simulink model "SimuOnlineComputeI1Level2C"  (R2024a)
settings: Solver=FixedStepAuto  StartTime=ti  StopTime=tf  FixedStep=Ts  RelTol=1e-3
settings Model: Creator=perruquetti  LastModifiedBy=perruquetti

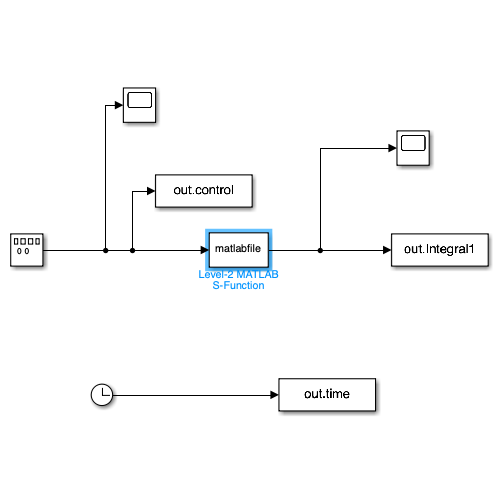
[thumbnail: Simulink's stored preview of the top-level diagram]
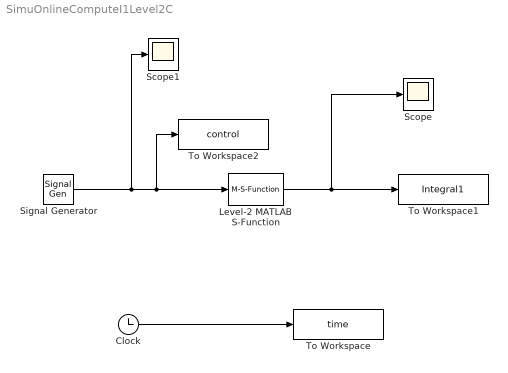
== system SimuOnlineComputeI1Level2C ==
  Clock : Clock
  Level-2 MATLAB S-Function : M-S-Function  Parameters=ParamI1
  Scope : Scope
  Scope1 : Scope
  Signal Generator : SignalGenerator  Units=rad/sec
  To Workspace : ToWorkspace  VariableName=time  SampleTime=-1
  To Workspace1 : ToWorkspace  VariableName=Integral1  SampleTime=-1
  To Workspace2 : ToWorkspace  VariableName=control  SampleTime=-1
  wires:
  Clock/1 -> To Workspace/1
  Level-2 MATLAB S-Function/1 -> Scope/1, To Workspace1/1
  Signal Generator/1 -> Scope1/1, Level-2 MATLAB S-Function/1, To Workspace2/1
